simulink model "acvh_tuner"  (R2020b)
settings: Solver=VariableStepAuto  StartTime=0.0  StopTime=100  RelTol=1e-3
model workspace (MAT data in the model file):
  Var = 0
values from neighbouring files (symbols this model uses):
  dragCoeffMov = 0.01    [iris_quadcopter_specs.m]
  g = 9.81    [iris_quadcopter_specs.m]
  inertia = diag([Ixx, Iyy, Izz])    [iris_quadcopter_specs.m]
  mass = 0.8    [iris_quadcopter_specs.m]
  rotorDir = [-1, -1, 1, 1]    [iris_quadcopter_specs.m]
  rotorPositions = zeros(3,4)    [iris_quadcopter_specs.m]
  rotorThrustMax = 4    [iris_quadcopter_specs.m]
  rotorTimeConst = 0.005    [iris_quadcopter_specs.m]
  rotorTorqueMax = 0.05    [iris_quadcopter_specs.m]
  SampleTime = 0.001    [iris_quadcopter_specs.m]
  windVel = [0 0 0]'    [iris_quadcopter_specs.m]
undefined symbols (not defined in the file or in its folder): dev, DiscIntNeverNeededParam, Main, pwm_output0
libraries: pid_lib x6, shared6dof x5, simulink x3, shared6dofsys x2, px4lib x1, sharedtransform x1, sharedutil x1, px4uORBlib x1
settings Model: EnablePacing=on  Creator=sid  LastModifiedBy=sid

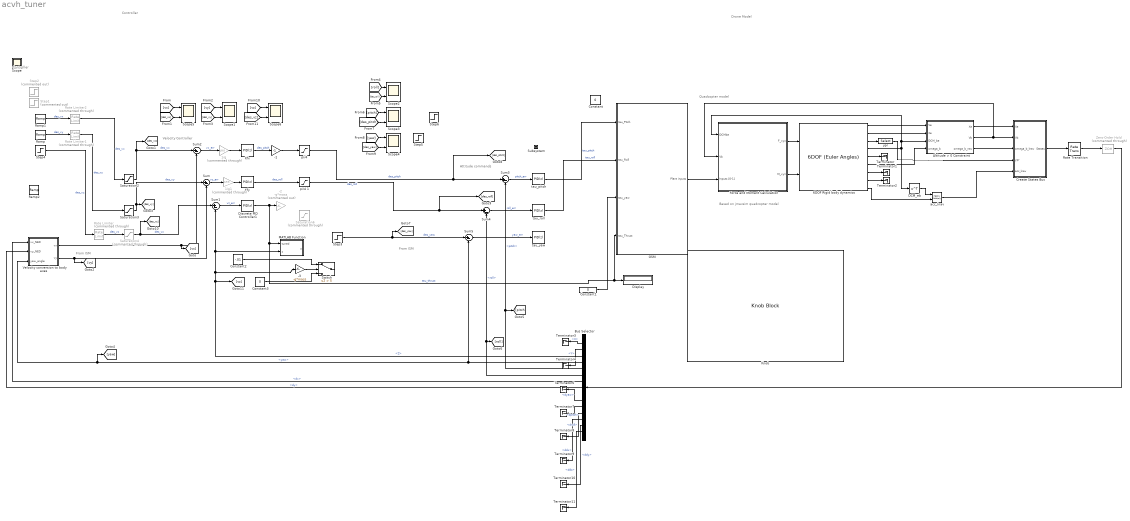
== system acvh_tuner ==
  note: Velocity Controller
  note: Attitude commands
  note: Controller
  note: Based on jmavsim quadcopter model
  note: Quadcopter model
  note: From ISM
  note: From ISM
  note: Controller
  note: Drone Model
  -1 : Gain  Gain=-1
  -2 : Gain  Commented=on  Gain=-g*mass
  -3 : Gain  Gain=-g*mass
  1/g : Gain  Commented=through  Gain=1/9.8
  1/g1 : Gain  Commented=through  Gain=1/9.8
  "6DOF Rigid body dynamics " : shared6dof/6DOF (Euler Angles)  units=Metric (MKS)  mtype=Fixed  rep=Euler Angles  xme_0=init.posNED  Vm_0=init.vb  eul_0=init.euler  pm_0=init.angRates  mass_0=mass  mass_e=0.5  mass_f=2.0  inertia=inertia  inertia_e=eye(3)  inertia_f=2*eye(3)  k_quat=Vehicle.SixDOF.quatGain  vre_flag=on  abi_flag=on  aMode=aMode  xme_statename=''  Vm_statename=''  eul_statename=''  quat_statename=''  pm_statename=''  mass_statename=''
      settings: SourceProductBaseCode=AE,PW,MT,UV,VE,VP
  Altitude > 0 Constraint : MATLAB Function  TreatAsAtomicUnit=on
  Bus Selector : BusSelector  OutputSignals=X,Y,Z,yaw,pitch,roll,dx,dy,dz,dyaw,dpitch,droll,ddx,ddy,ddz
  Constant : Constant  Value=0  SampleTime=SampleTime
  Constant1 : Constant  Value=0  SampleTime=SampleTime
  Constant2 : Constant  Value=-.01  SampleTime=SampleTime
  Constant3 : Constant  Value=0  SampleTime=SampleTime
  Create States Bus : Subsystem
  DCM_eb : Math  Operator=transpose  SaturateOnIntegerOverflow=on
  Discrete PID Controller1 : pid_lib/PID Controller  Controller=PID  Form=Parallel  TimeDomain=Discrete-time  UseExternalTs=off  SampleTime=SampleTime  IntegratorMethod=Trapezoidal  FilterMethod=Trapezoidal  ControllerParametersSource=internal  P=-0.0534535340221691  I=-0.00566953766767209  D=-0.123220888476467  UseFilter=on  N=26.3491959083223  TunerSelectOption=Transfer Function Based (PID Tuner App)  InitialConditionSource=internal  InitialConditionForIntegrator=0  InitialConditionForFilter=0  DifferentiatorICPrevScaledInput=0  ExternalReset=none  TrackingMode=off  Kt=1  LimitOutput=off  SatLimitsSource=internal  UpperSaturationLimit=10  LowerSaturationLimit=-.05  LinearizeAsGain=off  AntiWindupMode=back-calculation  Kb=10  POutMin=[]  POutMax=[]  IOutMin=[]  IOutMax=[]  DOutMin=[]  DOutMax=[]  NOutMin=[]  NOutMax=[]  SumOutMin=[]  SumOutMax=[]  SaturationOutMin=[]  SaturationOutMax=[]  PParamMin=[]  PParamMax=[]  IParamMin=[]  IParamMax=[]  DParamMin=[]  DParamMax=[]  NParamMin=[]  NParamMax=[]  KbParamMin=[]  KbParamMax=[]  KtParamMin=[]  KtParamMax=[]  KbOutMin=[]  KbOutMax=[]  KtOutMin=[]  KtOutMax=[]  IntegratorOutMin=[]  IntegratorOutMax=[]  FilterOutMin=[]  FilterOutMax=[]  SumI1OutMin=[]  SumI1OutMax=[]  SumI2OutMin=[]  SumI2OutMax=[]  SumI3OutMin=[]  SumI3OutMax=[]  SumI4OutMin=[]  SumI4OutMax=[]  SumDOutMin=[]  SumDOutMax=[]  DifferentiatorOutMin=[]  DifferentiatorOutMax=[]  FilterDiffOutCoefMin=[]  FilterDiffOutCoefMax=[]  ReciprocalOutMin=[]  ReciprocalOutMax=[]  SumDenOutMin=[]  SumDenOutMax=[]  SumNumOutMin=[]  SumNumOutMax=[]  DivideOutMin=[]  DivideOutMax=[]  UdiffTsProdOutMin=[]  UdiffTsProdOutMax=[]  NTsProdOutMin=[]  NTsProdOutMax=[]  UintegralTsProdOutMin=[]  UintegralTsProdOutMax=[]  UngainTsProdOutMin=[]  UngainTsProdOutMax=[]  IntegratorContinuousStateAttributes=''  IntegratorStateMustResolveToSignalObject=off  IntegratorRTWStateStorageClass=Auto  FilterContinuousStateAttributes=''  FilterStateMustResolveToSignalObject=off  FilterRTWStateStorageClass=Auto  ParallelPVariant=InternalParameters  IdealPVariant=Disabled  IVariant=InternalParameters  DVariant=InternalParameters  IntegratorVariant=Discrete  SatVariant=Disabled  AWVariant=Passthrough  PCopyVariant=Disabled  TRVariant=Disabled  FdbkBlocksVariant=Forward  IdealPFdbkVariant=Disabled  SatFdbkVariant=Disabled  DerivativeFilterVariant=TrapezoidalFilter  NVariant=InternalParameters  NCopyVariant=InternalParameters  FilterICVariant=InternalICsFilter  IntegratorICVariant=InternalICs  ExternalResetVariant=Disabled  TRSumVariant=Passthrough  SumFdbkVariant=Disabled  SumVariant=Sum_PID  TsampFilterVariant=InternalTs  TsampNgainVariant=Passthrough  TsampIntegralVariant=Passthrough  ExternalSaturationOutDataTypeStr=Inherit: Same as second input
  Display : Display
  Force and Moment Calculation : Subsystem
  Kfx : pid_lib/PID Controller  Controller=PID  Form=Parallel  TimeDomain=Discrete-time  UseExternalTs=off  SampleTime=SampleTime  IntegratorMethod=Forward Euler  FilterMethod=Forward Euler  ControllerParametersSource=internal  P=0.183358617742533  I=0.0739424315877928  D=-0.024031657470412  UseFilter=on  N=7.50922781087257  TunerSelectOption=Transfer Function Based (PID Tuner App)  InitialConditionSource=internal  InitialConditionForIntegrator=0  InitialConditionForFilter=0  DifferentiatorICPrevScaledInput=0  ExternalReset=none  TrackingMode=off  Kt=1  LimitOutput=on  SatLimitsSource=internal  UpperSaturationLimit=pi/8  LowerSaturationLimit=-pi/8  LinearizeAsGain=off  AntiWindupMode=clamping  Kb=1  POutMin=[]  POutMax=[]  IOutMin=[]  IOutMax=[]  DOutMin=[]  DOutMax=[]  NOutMin=[]  NOutMax=[]  SumOutMin=[]  SumOutMax=[]  SaturationOutMin=[]  SaturationOutMax=[]  PParamMin=[]  PParamMax=[]  IParamMin=[]  IParamMax=[]  DParamMin=[]  DParamMax=[]  NParamMin=[]  NParamMax=[]  KbParamMin=[]  KbParamMax=[]  KtParamMin=[]  KtParamMax=[]  KbOutMin=[]  KbOutMax=[]  KtOutMin=[]  KtOutMax=[]  IntegratorOutMin=[]  IntegratorOutMax=[]  FilterOutMin=[]  FilterOutMax=[]  SumI1OutMin=[]  SumI1OutMax=[]  SumI2OutMin=[]  SumI2OutMax=[]  SumI3OutMin=[]  SumI3OutMax=[]  SumI4OutMin=[]  SumI4OutMax=[]  SumDOutMin=[]  SumDOutMax=[]  DifferentiatorOutMin=[]  DifferentiatorOutMax=[]  FilterDiffOutCoefMin=[]  FilterDiffOutCoefMax=[]  ReciprocalOutMin=[]  ReciprocalOutMax=[]  SumDenOutMin=[]  SumDenOutMax=[]  SumNumOutMin=[]  SumNumOutMax=[]  DivideOutMin=[]  DivideOutMax=[]  UdiffTsProdOutMin=[]  UdiffTsProdOutMax=[]  NTsProdOutMin=[]  NTsProdOutMax=[]  UintegralTsProdOutMin=[]  UintegralTsProdOutMax=[]  UngainTsProdOutMin=[]  UngainTsProdOutMax=[]  IntegratorContinuousStateAttributes=''  IntegratorStateMustResolveToSignalObject=off  IntegratorRTWStateStorageClass=Auto  FilterContinuousStateAttributes=''  FilterStateMustResolveToSignalObject=off  FilterRTWStateStorageClass=Auto  ParallelPVariant=InternalParameters  IdealPVariant=Disabled  IVariant=InternalParameters  DVariant=InternalParameters  IntegratorVariant=Discrete  SatVariant=Enabled  AWVariant=DiscClampingParallel  PCopyVariant=Disabled  TRVariant=Disabled  FdbkBlocksVariant=Forward  IdealPFdbkVariant=Disabled  SatFdbkVariant=Disabled  DerivativeFilterVariant=ForwardEulerFilter  NVariant=InternalParameters  NCopyVariant=Disabled  FilterICVariant=InternalICsFilter  IntegratorICVariant=InternalICs  ExternalResetVariant=Disabled  TRSumVariant=Passthrough  SumFdbkVariant=Disabled  SumVariant=Sum_PID  TsampFilterVariant=InternalTs  TsampNgainVariant=Passthrough  TsampIntegralVariant=Passthrough  ExternalSaturationOutDataTypeStr=Inherit: Same as second input
  Kfy : pid_lib/PID Controller  Controller=PID  Form=Parallel  TimeDomain=Discrete-time  UseExternalTs=off  SampleTime=SampleTime  IntegratorMethod=Forward Euler  FilterMethod=Forward Euler  ControllerParametersSource=internal  P=0.183358617742446  I=0.0739424315877666  D=-0.0240316574704006  UseFilter=on  N=7.50922781087257  TunerSelectOption=Transfer Function Based (PID Tuner App)  InitialConditionSource=internal  InitialConditionForIntegrator=0  InitialConditionForFilter=0  DifferentiatorICPrevScaledInput=0  ExternalReset=none  TrackingMode=off  Kt=1  LimitOutput=on  SatLimitsSource=internal  UpperSaturationLimit=pi/8  LowerSaturationLimit=-pi/8  LinearizeAsGain=off  AntiWindupMode=clamping  Kb=1  POutMin=[]  POutMax=[]  IOutMin=[]  IOutMax=[]  DOutMin=[]  DOutMax=[]  NOutMin=[]  NOutMax=[]  SumOutMin=[]  SumOutMax=[]  SaturationOutMin=[]  SaturationOutMax=[]  PParamMin=[]  PParamMax=[]  IParamMin=[]  IParamMax=[]  DParamMin=[]  DParamMax=[]  NParamMin=[]  NParamMax=[]  KbParamMin=[]  KbParamMax=[]  KtParamMin=[]  KtParamMax=[]  KbOutMin=[]  KbOutMax=[]  KtOutMin=[]  KtOutMax=[]  IntegratorOutMin=[]  IntegratorOutMax=[]  FilterOutMin=[]  FilterOutMax=[]  SumI1OutMin=[]  SumI1OutMax=[]  SumI2OutMin=[]  SumI2OutMax=[]  SumI3OutMin=[]  SumI3OutMax=[]  SumI4OutMin=[]  SumI4OutMax=[]  SumDOutMin=[]  SumDOutMax=[]  DifferentiatorOutMin=[]  DifferentiatorOutMax=[]  FilterDiffOutCoefMin=[]  FilterDiffOutCoefMax=[]  ReciprocalOutMin=[]  ReciprocalOutMax=[]  SumDenOutMin=[]  SumDenOutMax=[]  SumNumOutMin=[]  SumNumOutMax=[]  DivideOutMin=[]  DivideOutMax=[]  UdiffTsProdOutMin=[]  UdiffTsProdOutMax=[]  NTsProdOutMin=[]  NTsProdOutMax=[]  UintegralTsProdOutMin=[]  UintegralTsProdOutMax=[]  UngainTsProdOutMin=[]  UngainTsProdOutMax=[]  IntegratorContinuousStateAttributes=''  IntegratorStateMustResolveToSignalObject=off  IntegratorRTWStateStorageClass=Auto  FilterContinuousStateAttributes=''  FilterStateMustResolveToSignalObject=off  FilterRTWStateStorageClass=Auto  ParallelPVariant=InternalParameters  IdealPVariant=Disabled  IVariant=InternalParameters  DVariant=InternalParameters  IntegratorVariant=Discrete  SatVariant=Enabled  AWVariant=DiscClampingParallel  PCopyVariant=Disabled  TRVariant=Disabled  FdbkBlocksVariant=Forward  IdealPFdbkVariant=Disabled  SatFdbkVariant=Disabled  DerivativeFilterVariant=ForwardEulerFilter  NVariant=InternalParameters  NCopyVariant=Disabled  FilterICVariant=InternalICsFilter  IntegratorICVariant=InternalICs  ExternalResetVariant=Disabled  TRSumVariant=Passthrough  SumFdbkVariant=Disabled  SumVariant=Sum_PID  TsampFilterVariant=InternalTs  TsampNgainVariant=Passthrough  TsampIntegralVariant=Passthrough  ExternalSaturationOutDataTypeStr=Inherit: Same as second input
  Knob : KnobBlock  ScaleMin=-1  ScaleMax=0
  MATLAB Function : MATLAB Function  TreatAsAtomicUnit=on
  OSM : Subsystem
  Ramp : simulink/Sources/Ramp  slope=3  start=10  InitialOutput=0
  Ramp1 : simulink/Sources/Ramp  slope=3  start=40  InitialOutput=0
  Ramp2 : simulink/Sources/Ramp  slope=-0.5  start=0  InitialOutput=-5
  Rate Limiter : RateLimiter  Commented=through  RisingSlewLimit=3  FallingSlewLimit=-3  SampleTimeMode=inherited  InitialCondition=-5
  Rate Limiter1 : RateLimiter  Commented=through  RisingSlewLimit=3  FallingSlewLimit=-3
  Rate Limiter2 : RateLimiter  Commented=through  RisingSlewLimit=3  FallingSlewLimit=-3
  Rate Transition : RateTransition  OutPortSampleTime=SampleTime
  Saturation2 : Saturate  UpperLimit=8  LowerLimit=-8  LinearizeAsGain=off
  Saturation3 : Saturate  UpperLimit=8  LowerLimit=-8  LinearizeAsGain=off
  Saturation4 : Saturate  Commented=through  UpperLimit=1  LowerLimit=-6
  Saturation6 : Saturate  Commented=through  UpperLimit=.12*g*mass  LowerLimit=-5*g*mass  SampleTime=SampleTime
  Scope{1..6} (6 alike) : Scope  NumInputPorts=2
  Step1 : Step  Commented=on  Time=40  SampleTime=SampleTime
  Step2 : Step  Commented=on  Time=10  SampleTime=SampleTime
  Step3 : Step  SampleTime=SampleTime
  Step4 : Step  Before=-5  After=-6  SampleTime=SampleTime
  Step5 : Step  After=pi/5  SampleTime=SampleTime
  Step6 : Step  After=pi/5  SampleTime=SampleTime
  Subsystem : Subsystem
  Sum{,1..5} (6 alike) : Sum  Inputs=|+-
  Switch : Switch  Criteria=u2 > Threshold  Threshold=5
  Terminator{,1..4,6..11} (11 alike) : Terminator
  Velocity conversion to body axes : Subsystem
  Zero-Order Hold : ZeroOrderHold  Commented=through  SampleTime=SampleTime
  acc_lnav : Product  Multiplication=Matrix(*)
  pi/4 : Saturate  UpperLimit=pi/4  LowerLimit=-pi/4
  pi/4 1 : Saturate  UpperLimit=pi/4  LowerLimit=-pi/4
  tau_pitch : pid_lib/PID Controller  Controller=PID  Form=Parallel  TimeDomain=Discrete-time  UseExternalTs=off  SampleTime=SampleTime  IntegratorMethod=Forward Euler  FilterMethod=Forward Euler  ControllerParametersSource=internal  P=0.0543673511512337  I=0.0109980209644375  D=0.0263229670839572  UseFilter=on  N=347.83750102845  TunerSelectOption=Transfer Function Based (PID Tuner App)  InitialConditionSource=internal  InitialConditionForIntegrator=0  InitialConditionForFilter=0  DifferentiatorICPrevScaledInput=0  ExternalReset=none  TrackingMode=off  Kt=1  LimitOutput=on  SatLimitsSource=internal  UpperSaturationLimit=.05  LowerSaturationLimit=-.05  LinearizeAsGain=off  AntiWindupMode=none  Kb=1  POutMin=[]  POutMax=[]  IOutMin=[]  IOutMax=[]  DOutMin=[]  DOutMax=[]  NOutMin=[]  NOutMax=[]  SumOutMin=[]  SumOutMax=[]  SaturationOutMin=[]  SaturationOutMax=[]  PParamMin=[]  PParamMax=[]  IParamMin=[]  IParamMax=[]  DParamMin=[]  DParamMax=[]  NParamMin=[]  NParamMax=[]  KbParamMin=[]  KbParamMax=[]  KtParamMin=[]  KtParamMax=[]  KbOutMin=[]  KbOutMax=[]  KtOutMin=[]  KtOutMax=[]  IntegratorOutMin=[]  IntegratorOutMax=[]  FilterOutMin=[]  FilterOutMax=[]  SumI1OutMin=[]  SumI1OutMax=[]  SumI2OutMin=[]  SumI2OutMax=[]  SumI3OutMin=[]  SumI3OutMax=[]  SumI4OutMin=[]  SumI4OutMax=[]  SumDOutMin=[]  SumDOutMax=[]  DifferentiatorOutMin=[]  DifferentiatorOutMax=[]  FilterDiffOutCoefMin=[]  FilterDiffOutCoefMax=[]  ReciprocalOutMin=[]  ReciprocalOutMax=[]  SumDenOutMin=[]  SumDenOutMax=[]  SumNumOutMin=[]  SumNumOutMax=[]  DivideOutMin=[]  DivideOutMax=[]  UdiffTsProdOutMin=[]  UdiffTsProdOutMax=[]  NTsProdOutMin=[]  NTsProdOutMax=[]  UintegralTsProdOutMin=[]  UintegralTsProdOutMax=[]  UngainTsProdOutMin=[]  UngainTsProdOutMax=[]  IntegratorContinuousStateAttributes=''  IntegratorStateMustResolveToSignalObject=off  IntegratorRTWStateStorageClass=Auto  FilterContinuousStateAttributes=''  FilterStateMustResolveToSignalObject=off  FilterRTWStateStorageClass=Auto  ParallelPVariant=InternalParameters  IdealPVariant=Disabled  IVariant=InternalParameters  DVariant=InternalParameters  IntegratorVariant=Discrete  SatVariant=Enabled  AWVariant=Passthrough  PCopyVariant=Disabled  TRVariant=Disabled  FdbkBlocksVariant=Forward  IdealPFdbkVariant=Disabled  SatFdbkVariant=Disabled  DerivativeFilterVariant=ForwardEulerFilter  NVariant=InternalParameters  NCopyVariant=Disabled  FilterICVariant=InternalICsFilter  IntegratorICVariant=InternalICs  ExternalResetVariant=Disabled  TRSumVariant=Passthrough  SumFdbkVariant=Disabled  SumVariant=Sum_PID  TsampFilterVariant=InternalTs  TsampNgainVariant=Passthrough  TsampIntegralVariant=Passthrough  ExternalSaturationOutDataTypeStr=Inherit: Same as second input
  tau_roll : pid_lib/PID Controller  Controller=PID  Form=Parallel  TimeDomain=Discrete-time  UseExternalTs=off  SampleTime=SampleTime  IntegratorMethod=Forward Euler  FilterMethod=Forward Euler  ControllerParametersSource=internal  P=-0.0543673511512337  I=-0.0109980209644375  D=-0.0263229670839572  UseFilter=on  N=347.83750102845  TunerSelectOption=Transfer Function Based (PID Tuner App)  InitialConditionSource=internal  InitialConditionForIntegrator=0  InitialConditionForFilter=0  DifferentiatorICPrevScaledInput=0  ExternalReset=none  TrackingMode=off  Kt=1  LimitOutput=on  SatLimitsSource=internal  UpperSaturationLimit=.05  LowerSaturationLimit=-.05  LinearizeAsGain=off  AntiWindupMode=none  Kb=1  POutMin=[]  POutMax=[]  IOutMin=[]  IOutMax=[]  DOutMin=[]  DOutMax=[]  NOutMin=[]  NOutMax=[]  SumOutMin=[]  SumOutMax=[]  SaturationOutMin=[]  SaturationOutMax=[]  PParamMin=[]  PParamMax=[]  IParamMin=[]  IParamMax=[]  DParamMin=[]  DParamMax=[]  NParamMin=[]  NParamMax=[]  KbParamMin=[]  KbParamMax=[]  KtParamMin=[]  KtParamMax=[]  KbOutMin=[]  KbOutMax=[]  KtOutMin=[]  KtOutMax=[]  IntegratorOutMin=[]  IntegratorOutMax=[]  FilterOutMin=[]  FilterOutMax=[]  SumI1OutMin=[]  SumI1OutMax=[]  SumI2OutMin=[]  SumI2OutMax=[]  SumI3OutMin=[]  SumI3OutMax=[]  SumI4OutMin=[]  SumI4OutMax=[]  SumDOutMin=[]  SumDOutMax=[]  DifferentiatorOutMin=[]  DifferentiatorOutMax=[]  FilterDiffOutCoefMin=[]  FilterDiffOutCoefMax=[]  ReciprocalOutMin=[]  ReciprocalOutMax=[]  SumDenOutMin=[]  SumDenOutMax=[]  SumNumOutMin=[]  SumNumOutMax=[]  DivideOutMin=[]  DivideOutMax=[]  UdiffTsProdOutMin=[]  UdiffTsProdOutMax=[]  NTsProdOutMin=[]  NTsProdOutMax=[]  UintegralTsProdOutMin=[]  UintegralTsProdOutMax=[]  UngainTsProdOutMin=[]  UngainTsProdOutMax=[]  IntegratorContinuousStateAttributes=''  IntegratorStateMustResolveToSignalObject=off  IntegratorRTWStateStorageClass=Auto  FilterContinuousStateAttributes=''  FilterStateMustResolveToSignalObject=off  FilterRTWStateStorageClass=Auto  ParallelPVariant=InternalParameters  IdealPVariant=Disabled  IVariant=InternalParameters  DVariant=InternalParameters  IntegratorVariant=Discrete  SatVariant=Enabled  AWVariant=Passthrough  PCopyVariant=Disabled  TRVariant=Disabled  FdbkBlocksVariant=Forward  IdealPFdbkVariant=Disabled  SatFdbkVariant=Disabled  DerivativeFilterVariant=ForwardEulerFilter  NVariant=InternalParameters  NCopyVariant=Disabled  FilterICVariant=InternalICsFilter  IntegratorICVariant=InternalICs  ExternalResetVariant=Disabled  TRSumVariant=Passthrough  SumFdbkVariant=Disabled  SumVariant=Sum_PID  TsampFilterVariant=InternalTs  TsampNgainVariant=Passthrough  TsampIntegralVariant=Passthrough  ExternalSaturationOutDataTypeStr=Inherit: Same as second input
  tau_yaw : pid_lib/PID Controller  Controller=PID  Form=Parallel  TimeDomain=Discrete-time  UseExternalTs=off  SampleTime=SampleTime  IntegratorMethod=Forward Euler  FilterMethod=Forward Euler  ControllerParametersSource=internal  P=-0.564155915391973  I=-0.130215223566003  D=-0.447814603729917  UseFilter=on  N=347.83750102845  TunerSelectOption=Transfer Function Based (PID Tuner App)  InitialConditionSource=internal  InitialConditionForIntegrator=0  InitialConditionForFilter=0  DifferentiatorICPrevScaledInput=0  ExternalReset=none  TrackingMode=off  Kt=1  LimitOutput=on  SatLimitsSource=internal  UpperSaturationLimit=0.1  LowerSaturationLimit=-0.1  LinearizeAsGain=off  AntiWindupMode=none  Kb=1  POutMin=[]  POutMax=[]  IOutMin=[]  IOutMax=[]  DOutMin=[]  DOutMax=[]  NOutMin=[]  NOutMax=[]  SumOutMin=[]  SumOutMax=[]  SaturationOutMin=[]  SaturationOutMax=[]  PParamMin=[]  PParamMax=[]  IParamMin=[]  IParamMax=[]  DParamMin=[]  DParamMax=[]  NParamMin=[]  NParamMax=[]  KbParamMin=[]  KbParamMax=[]  KtParamMin=[]  KtParamMax=[]  KbOutMin=[]  KbOutMax=[]  KtOutMin=[]  KtOutMax=[]  IntegratorOutMin=[]  IntegratorOutMax=[]  FilterOutMin=[]  FilterOutMax=[]  SumI1OutMin=[]  SumI1OutMax=[]  SumI2OutMin=[]  SumI2OutMax=[]  SumI3OutMin=[]  SumI3OutMax=[]  SumI4OutMin=[]  SumI4OutMax=[]  SumDOutMin=[]  SumDOutMax=[]  DifferentiatorOutMin=[]  DifferentiatorOutMax=[]  FilterDiffOutCoefMin=[]  FilterDiffOutCoefMax=[]  ReciprocalOutMin=[]  ReciprocalOutMax=[]  SumDenOutMin=[]  SumDenOutMax=[]  SumNumOutMin=[]  SumNumOutMax=[]  DivideOutMin=[]  DivideOutMax=[]  UdiffTsProdOutMin=[]  UdiffTsProdOutMax=[]  NTsProdOutMin=[]  NTsProdOutMax=[]  UintegralTsProdOutMin=[]  UintegralTsProdOutMax=[]  UngainTsProdOutMin=[]  UngainTsProdOutMax=[]  IntegratorContinuousStateAttributes=''  IntegratorStateMustResolveToSignalObject=off  IntegratorRTWStateStorageClass=Auto  FilterContinuousStateAttributes=''  FilterStateMustResolveToSignalObject=off  FilterRTWStateStorageClass=Auto  ParallelPVariant=InternalParameters  IdealPVariant=Disabled  IVariant=InternalParameters  DVariant=InternalParameters  IntegratorVariant=Discrete  SatVariant=Enabled  AWVariant=Passthrough  PCopyVariant=Disabled  TRVariant=Disabled  FdbkBlocksVariant=Forward  IdealPFdbkVariant=Disabled  SatFdbkVariant=Disabled  DerivativeFilterVariant=ForwardEulerFilter  NVariant=InternalParameters  NCopyVariant=Disabled  FilterICVariant=InternalICsFilter  IntegratorICVariant=InternalICs  ExternalResetVariant=Disabled  TRSumVariant=Passthrough  SumFdbkVariant=Disabled  SumVariant=Sum_PID  TsampFilterVariant=InternalTs  TsampNgainVariant=Passthrough  TsampIntegralVariant=Passthrough  ExternalSaturationOutDataTypeStr=Inherit: Same as second input
  ypr : Selector  InputPortWidth=3  IndexOptions=Index vector (dialog)  Indices=[3 2 1]  OutputSizes=1
  Scope : Scope
  wires:
  "6DOF Rigid body dynamics "/6 -> Altitude > 0 Constraint/4(omega_b)
  Altitude > 0 Constraint/1(Xe) -> Create States Bus/1(Xe)
  "6DOF Rigid body dynamics "/1 -> Altitude > 0 Constraint/1(Ve)
  "6DOF Rigid body dynamics "/2 -> Altitude > 0 Constraint/2("Xe ")
  "6DOF Rigid body dynamics "/3 -> ypr/1
  acc_lnav/1 -> Create States Bus/5(acc_lnav)
  "6DOF Rigid body dynamics "/5 -> Terminator/1
  Altitude > 0 Constraint/3(omega_b_nav) -> Create States Bus/3(omega_b_lnav)
  "6DOF Rigid body dynamics "/9 -> acc_lnav/2
  "6DOF Rigid body dynamics "/4 -> DCM_eb/1, Force and Moment Calculation/1(DCMbe), Altitude > 0 Constraint/3(DCM_be)
  DCM_eb/1 -> acc_lnav/1
  Force and Moment Calculation/2(M_xyz) -> "6DOF Rigid body dynamics "/2
  "6DOF Rigid body dynamics "/7 -> Terminator1/1
  "6DOF Rigid body dynamics "/8 -> Terminator2/1
  Force and Moment Calculation/1(F_xyz) -> "6DOF Rigid body dynamics "/1
  Create States Bus/1(States) -> Rate Transition/1
  ypr/1 -> Create States Bus/4(ypr)
  OSM/1(Plant inputs) -> Force and Moment Calculation/3(Inputs [0-1])
  Altitude > 0 Constraint/2(Vb) -> Force and Moment Calculation/2(Vb), Create States Bus/2(Vb)
  Zero-Order Hold/1 -> Bus Selector/1
  Bus Selector/1 -> Terminator3/1  "<X>"
  Bus Selector/2 -> Terminator4/1  "<Y>"
  Bus Selector/4 -> [yaw], Velocity conversion to body axes/3(yaw_angle), Sum5/2  "<yaw>"
  Bus Selector/5 -> [pitch], Sum3/2  "<pitch>"
  Bus Selector/6 -> Sum4/2, [roll]  "<roll>"
  Bus Selector/7 -> Velocity conversion to body axes/1(vx_NED)  "<dx>"
  Bus Selector/8 -> Velocity conversion to body axes/2(vy_NED)  "<dy>"
  Bus Selector/10 -> Terminator6/1  "<dyaw>"
  Bus Selector/11 -> Terminator7/1  "<dpitch>"
  Bus Selector/12 -> Terminator8/1  "<droll>"
  Bus Selector/13 -> Terminator9/1  "<ddx>"
  Bus Selector/14 -> Terminator10/1  "<ddy>"
  Bus Selector/15 -> Terminator11/1  "<ddz>"
  Rate Transition/1 -> Zero-Order Hold/1
  [des_yaw] -> Scope4/2
  [yaw] -> Scope4/1
  [des_pitch] -> Scope3/2
  [pitch] -> Scope3/1
  [des_roll] -> Scope2/2
  [roll] -> Scope2/1
  [des_vy] -> Scope1/2
  [vy] -> Scope1/1
  [des_vx] -> Scope5/2
  [vx] -> Scope5/1
  Step4/1 -> Rate Limiter/1  "des_vz"
  Sum3/1 -> tau_pitch/1  "pitch_err"
  Sum4/1 -> tau_roll/1  "roll_err"
  Sum5/1 -> tau_yaw/1  "yaw_err"
  Step3/1 -> [des_yaw], Sum5/1  "des_yaw"
  1/g1/1 -> Kfy/1
  1/g/1 -> Kfx/1
  Discrete PID Controller1/1 -> OSM/4(tau_Thrust), Display/1, MATLAB Function/1(tuned), -2/1  "tau_thrust"
  Velocity conversion to body axes/2(vy) -> Sum/2, [vy]
  Kfx/1 -> -1/1  "des_pitch"
  Saturation2/1 -> Sum2/1, [des_vx]  "des_vx"
  Velocity conversion to body axes/1(vx) -> Sum2/2, [vx]
  Sum/1 -> 1/g1/1  "vy_err"
  Saturation3/1 -> Sum/1, [des_vy]  "des_vy"
  Kfy/1 -> pi/4 1/1  "des_roll"
  Sum1/1 -> Discrete PID Controller1/1  "vz_err"
  Sum2/1 -> 1/g/1  "vx_err"
  -1/1 -> pi/4/1
  [vz] -> Scope6/1
  [des_vz] -> Scope6/2
  ? -> Subsystem/Trigger
  ? -> Subsystem/1(In1)
  pi/4/1 -> [des_pitch], Sum3/1  "des_pitch"
  pi/4 1/1 -> [des_roll], Sum4/1  "des_roll"
  Bus Selector/3 -> MATLAB Function/2(z), Sum1/2, -3/1, [vz]  "<Z>"
  Constant1/1 -> OSM/3(tau_yaw)
  Saturation4/1 -> Sum1/1, [des_vz]  "des_vz"
  tau_pitch/1 -> OSM/1(tau_Pitch)  "tau_pitch"
  tau_roll/1 -> OSM/2(tau_Roll)  "tau_roll"
  Rate Limiter/1 -> Saturation4/1  "des_vz"
  Rate Limiter1/1 -> Saturation3/1  "des_vy"
  Rate Limiter2/1 -> Saturation2/1  "des_vx"
  Ramp1/1 -> Rate Limiter2/1  "des_vx"
  Ramp/1 -> Rate Limiter1/1  "des_vy"
  -3/1 -> Switch/2
  Constant2/1 -> Switch/1
  Constant3/1 -> Switch/3

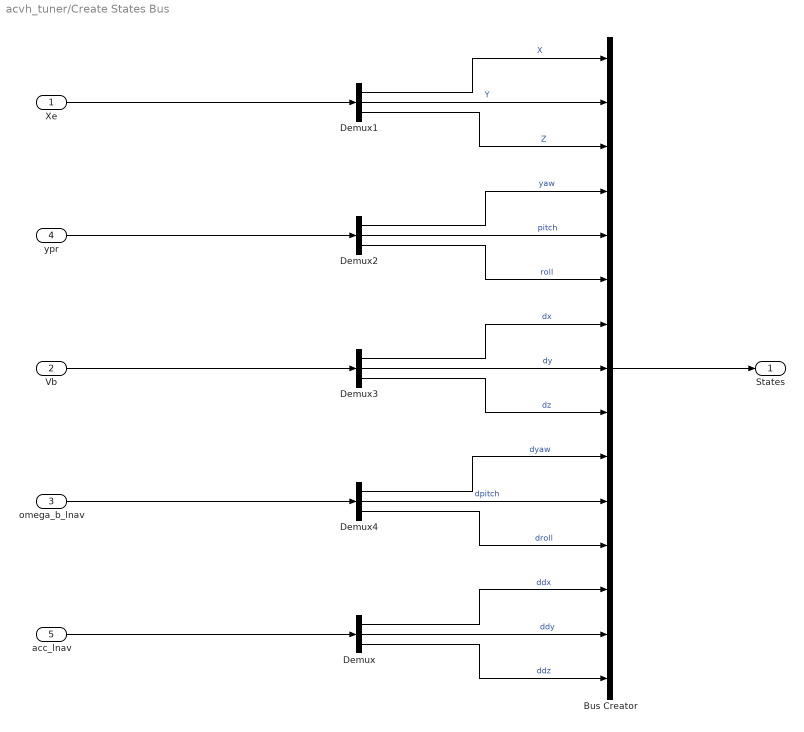
== system acvh_tuner/Create States Bus ==
  Xe : Inport
  Vb : Inport  Port=2
  omega_b_lnav : Inport  Port=3
  ypr : Inport  Port=4
  acc_lnav : Inport  Port=5
  Bus Creator : BusCreator  Inputs=15
  Demux{,1..4} (5 alike) : Demux  Outputs=3
  States : Outport
  wires:
  Demux1/1 -> Bus Creator/1  "X"
  Demux1/2 -> Bus Creator/2  "Y"
  ypr/1 -> Demux2/1
  Demux2/2 -> Bus Creator/5  "pitch"
  Demux3/2 -> Bus Creator/8  "dy"
  Demux2/3 -> Bus Creator/6  "roll"
  omega_b_lnav/1 -> Demux4/1
  Vb/1 -> Demux3/1
  Demux2/1 -> Bus Creator/4  "yaw"
  Demux1/3 -> Bus Creator/3  "Z"
  Demux3/1 -> Bus Creator/7  "dx"
  Demux4/2 -> Bus Creator/11  "dpitch"
  Demux3/3 -> Bus Creator/9  "dz"
  Demux4/3 -> Bus Creator/12  "droll"
  Demux4/1 -> Bus Creator/10  "dyaw"
  Bus Creator/1 -> States/1
  Xe/1 -> Demux1/1
  acc_lnav/1 -> Demux/1
  Demux/3 -> Bus Creator/15  "ddz"
  Demux/2 -> Bus Creator/14  "ddy"
  Demux/1 -> Bus Creator/13  "ddx"

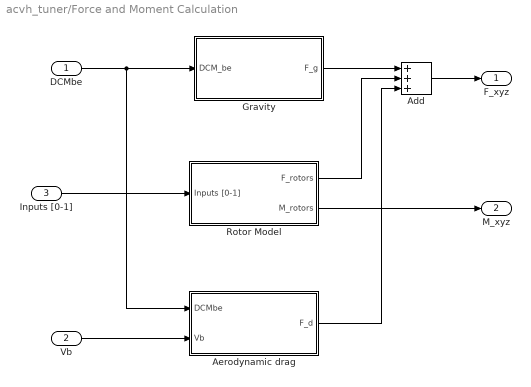
== system acvh_tuner/Force and Moment Calculation ==
  DCMbe : Inport
  Vb : Inport  Port=2
  Inputs [0-1] : Inport  Port=3
  Add : Sum  Inputs=+++
  Aerodynamic drag : Subsystem
  Gravity : Subsystem
  Rotor Model : Subsystem
  F_xyz : Outport
  M_xyz : Outport  Port=2
  wires:
  Inputs [0-1]/1 -> Rotor Model/1(Inputs [0-1])
  DCMbe/1 -> Aerodynamic drag/1(DCMbe), Gravity/1(DCM_be)
  Gravity/1(F_g) -> Add/1
  Add/1 -> F_xyz/1
  Rotor Model/2(M_rotors) -> M_xyz/1
  Vb/1 -> Aerodynamic drag/2(Vb)
  Rotor Model/1(F_rotors) -> Add/2
  Aerodynamic drag/1(F_d) -> Add/3

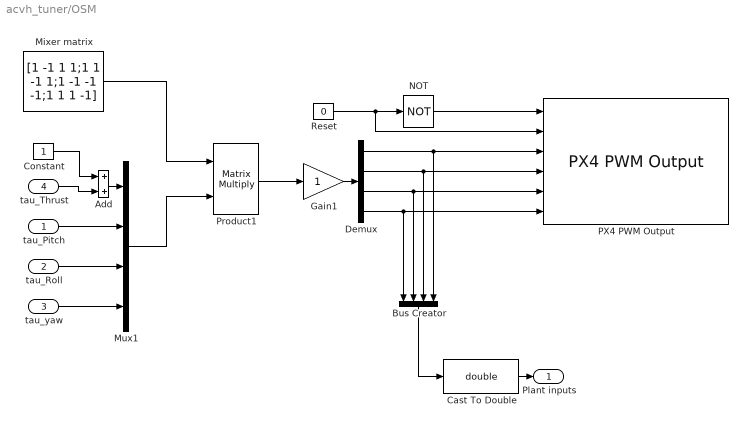
== system acvh_tuner/OSM ==
  tau_Pitch : Inport
  tau_Roll : Inport  Port=2
  tau_yaw : Inport  Port=3
  tau_Thrust : Inport  Port=4
  Add : Sum
  Bus Creator : BusCreator  Inputs=4
  Cast To Double : DataTypeConversion  OutDataTypeStr=double
  Constant : Constant  SampleTime=SampleTime
  Demux : Demux
  Gain1 : Gain  OutDataTypeStr=uint16
  Mixer matrix : Constant  Value=[1 -1 1 1;1 1 -1 1;1 -1 -1 -1;1 1 1 -1]  OutDataTypeStr=Inherit: Inherit via back propagation
  Mux1 : Mux
  NOT : Logic  Operator=NOT  IconShape=distinctive  AllPortsSameDT=off  OutDataTypeStr=boolean
  PX4 PWM Output : px4lib/PX4 PWM Output  pwmDevice=Main (/dev/pwm_output0)  pwmChannel1_=on  pwmChannel2_=on  pwmChannel3_=on  pwmChannel4_=on  pwmChannel5_=off  pwmChannel6_=off  pwmChannel7_=off  pwmChannel8_=off  forceTerminateFailsafe=off  outputErrorStatus=off
      settings: SourceProductBaseCode=PX4AUTOPILOTS
  Product1 : Product  Multiplication=Matrix(*)  RndMeth=Zero
  Reset : Constant  Value=0  OutDataTypeStr=boolean
  Plant inputs : Outport
  wires:
  NOT/1 -> PX4 PWM Output/1
  Mixer matrix/1 -> Product1/1
  tau_yaw/1 -> Mux1/4
  tau_Pitch/1 -> Mux1/2
  tau_Roll/1 -> Mux1/3
  Reset/1 -> PX4 PWM Output/2, NOT/1
  Demux/3 -> Bus Creator/2, PX4 PWM Output/5
  Demux/2 -> Bus Creator/3, PX4 PWM Output/4
  Mux1/1 -> Product1/2
  Demux/4 -> Bus Creator/1, PX4 PWM Output/6
  Gain1/1 -> Demux/1
  Demux/1 -> Bus Creator/4, PX4 PWM Output/3
  Product1/1 -> Gain1/1
  tau_Thrust/1 -> Add/2
  Add/1 -> Mux1/1
  Constant/1 -> Add/1
  Cast To Double/1 -> Plant inputs/1
  Bus Creator/1 -> Cast To Double/1

== system acvh_tuner/Subsystem ==
  In1 : Inport
  Trigger : TriggerPort  VariantControl=Variant  PortDimensions=1
  6DOF Rigid Body Dynamics : Subsystem  Commented=on
  Commands : Subsystem  Commented=on

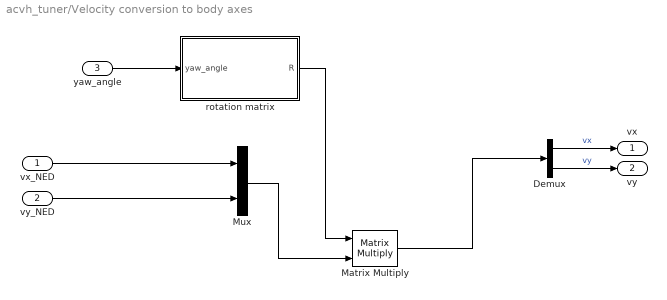
== system acvh_tuner/Velocity conversion to body axes ==
  vx_NED : Inport
  vy_NED : Inport  Port=2
  yaw_angle : Inport  Port=3
  Demux : Demux  Outputs=2
  Matrix Multiply : Product  Multiplication=Matrix(*)
  Mux : Mux  Inputs=2
  rotation matrix : Subsystem
  vx : Outport
  vy : Outport  Port=2
  wires:
  vy_NED/1 -> Mux/2
  vx_NED/1 -> Mux/1
  Demux/1 -> vx/1  "vx"
  Demux/2 -> vy/1  "vy"
  rotation matrix/1(R) -> Matrix Multiply/1
  Matrix Multiply/1 -> Demux/1
  yaw_angle/1 -> rotation matrix/1(yaw_angle)
  Mux/1 -> Matrix Multiply/2

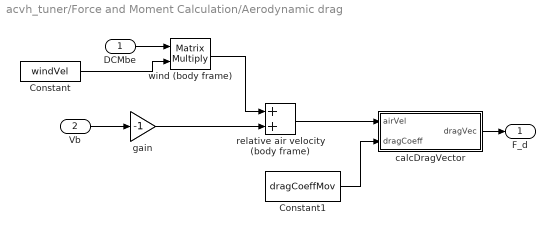
== system acvh_tuner/Force and Moment Calculation/Aerodynamic drag ==
  DCMbe : Inport
  Vb : Inport  Port=2
  Constant : Constant  Value=windVel  SampleTime=SampleTime
  Constant1 : Constant  Value=dragCoeffMov  SampleTime=SampleTime
  calcDragVector : MATLAB Function  TreatAsAtomicUnit=on
  gain : Gain  Gain=-1
  relative air velocity (body frame) : Sum
  wind (body frame) : Product  Multiplication=Matrix(*)
  F_d : Outport
  wires:
  Vb/1 -> gain/1
  calcDragVector/1(dragVec) -> F_d/1
  relative air velocity (body frame)/1 -> calcDragVector/1(airVel)
  gain/1 -> relative air velocity (body frame)/2
  Constant1/1 -> calcDragVector/2(dragCoeff)
  DCMbe/1 -> wind (body frame)/1
  Constant/1 -> wind (body frame)/2
  wind (body frame)/1 -> relative air velocity (body frame)/1

== system acvh_tuner/Force and Moment Calculation/Gravity ==
  DCM_be : Inport
  Constant : Constant  Value=[0 0 g]'
  Gain : Gain  Gain=mass
  Matrix Multiply : Product  Multiplication=Matrix(*)
  F_g : Outport
  wires:
  Matrix Multiply/1 -> Gain/1
  Constant/1 -> Matrix Multiply/2
  DCM_be/1 -> Matrix Multiply/1
  Gain/1 -> F_g/1

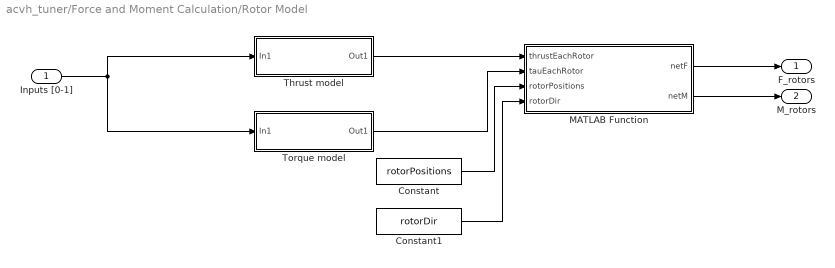
== system acvh_tuner/Force and Moment Calculation/Rotor Model ==
  Inputs [0-1] : Inport
  Constant : Constant  Value=rotorPositions
  Constant1 : Constant  Value=rotorDir
  MATLAB Function : MATLAB Function  TreatAsAtomicUnit=on
  Thrust model : Subsystem
  Torque model : Subsystem
  F_rotors : Outport
  M_rotors : Outport  Port=2
  wires:
  Inputs [0-1]/1 -> Torque model/1(In1), Thrust model/1(In1)
  MATLAB Function/1(netF) -> F_rotors/1
  MATLAB Function/2(netM) -> M_rotors/1
  Constant/1 -> MATLAB Function/3(rotorPositions)
  Constant1/1 -> MATLAB Function/4(rotorDir)
  Torque model/1(Out1) -> MATLAB Function/2(tauEachRotor)
  Thrust model/1(Out1) -> MATLAB Function/1(thrustEachRotor)

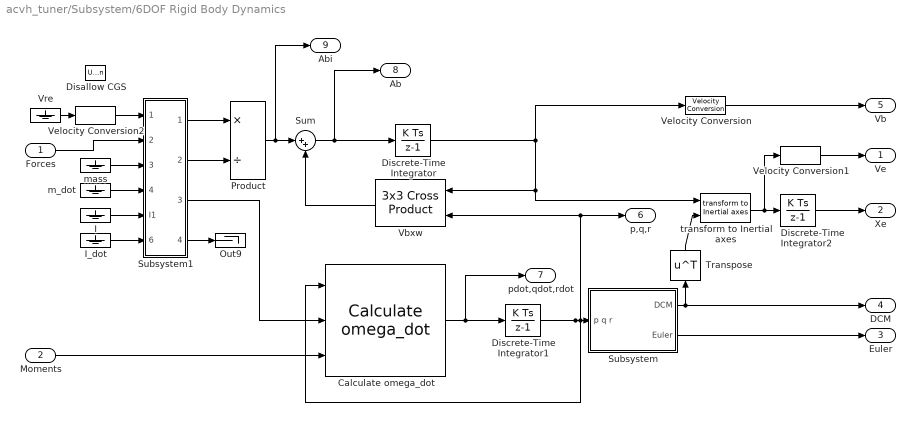
== system acvh_tuner/Subsystem/6DOF Rigid Body Dynamics ==
  Forces : Inport  Unit=N  PortDimensions=3
  Moments : Inport  Port=2  Unit=N*m  PortDimensions=3
  Calculate omega_dot : shared6dofsys/Calculate omega_dot  aMode=aMode
      settings: SourceProductBaseCode=AE,PW,MT,UV,VE,VP
  Disallow CGS : UnitConfiguration  UnitSystemsStr=English,SI,SI (extended)  AllowAllUnitSystems=off
  Discrete-Time Integrator : DiscreteIntegrator  SampleTime=SampleTime  ICPrevOutput=DiscIntNeverNeededParam  ICPrevScaledInput=DiscIntNeverNeededParam
  Discrete-Time Integrator1 : DiscreteIntegrator  SampleTime=SampleTime  ICPrevOutput=DiscIntNeverNeededParam  ICPrevScaledInput=DiscIntNeverNeededParam
  Discrete-Time Integrator2 : DiscreteIntegrator  SampleTime=SampleTime  ICPrevOutput=DiscIntNeverNeededParam  ICPrevScaledInput=DiscIntNeverNeededParam
  I : Ground
  I_dot : Ground
  Out9 : Terminator
  Product : Product  Inputs=*/  SaturateOnIntegerOverflow=on  OutDataTypeStr=Inherit: Same as first input
  Subsystem : Subsystem
  Subsystem1 : Subsystem
  Sum : Sum  Inputs=|++  SaturateOnIntegerOverflow=on
  Transpose : Math  Operator=transpose  SignedPower=on  SaturateOnIntegerOverflow=on
  Vbxw : sharedutil/3x3 Cross Product  aMode=aMode
      settings: SourceProductBaseCode=AE,PW,MT,UV,VE,VP
  Velocity Conversion : shared6dof/6DOF (Euler Angles)/Velocity Conversion  SystemSampleTime=-1  VariantActivationTime=update diagram  Latency=0  AutoFrameSizeCalculation=off
      settings: SourceProductBaseCode=AE,PW,MT,UV,VE,VP
  Velocity Conversion1 : shared6dof/6DOF (Euler Angles)/Velocity Conversion1  SystemSampleTime=-1  VariantActivationTime=update diagram  Latency=0  AutoFrameSizeCalculation=off
      settings: SourceProductBaseCode=AE,PW,MT,UV,VE,VP
  Velocity Conversion2 : shared6dof/6DOF (Euler Angles)/Velocity Conversion2  SystemSampleTime=-1  VariantActivationTime=update diagram  Latency=0  AutoFrameSizeCalculation=off
      settings: SourceProductBaseCode=AE,PW,MT,UV,VE,VP
  Vre : Ground
  m_dot : Ground
  mass : Ground
  "transform to Inertial axes " : shared6dof/6DOF (Euler Angles)/transform to Inertial axes   SystemSampleTime=-1  VariantActivationTime=update diagram  Latency=0  AutoFrameSizeCalculation=off
      settings: SourceProductBaseCode=AE,PW,MT,UV,VE,VP
  Ve : Outport  Unit=m/s  VectorParamsAs1DForOutWhenUnconnected=off
  Xe : Outport  Port=2  Unit=m  VectorParamsAs1DForOutWhenUnconnected=off
  Euler : Outport  Port=3  Unit=rad  VectorParamsAs1DForOutWhenUnconnected=off
  DCM : Outport  Port=4  Unit=1  VectorParamsAs1DForOutWhenUnconnected=off
  Vb : Outport  Port=5  Unit=m/s  VectorParamsAs1DForOutWhenUnconnected=off
  p,q,r : Outport  Port=6  Unit=rad/s  VectorParamsAs1DForOutWhenUnconnected=off
  pdot,qdot,rdot : Outport  Port=7  Unit=rad/s^2  VectorParamsAs1DForOutWhenUnconnected=off
  Ab : Outport  Port=8  Unit=m/s^2  VectorParamsAs1DForOutWhenUnconnected=off
  Abi : Outport  Port=9  Unit=m/s^2
  wires:
  mass/1 -> Subsystem1/3("mass ")
  Subsystem1/4(Out1) -> Out9/1
  Forces/1 -> Subsystem1/2(forces)
  Transpose/1 -> "transform to Inertial axes "/2
  Discrete-Time Integrator1/1 -> Calculate omega_dot/1, p,q,r/1, Vbxw/2, Subsystem/1("p q r ")
  Subsystem1/1("forces ") -> Product/1
  Discrete-Time Integrator2/1 -> Xe/1
  Vbxw/1 -> Sum/2
  "transform to Inertial axes "/1 -> Velocity Conversion1/1, Discrete-Time Integrator2/1
  Subsystem1/2(mass1) -> Product/2
  Velocity Conversion2/1 -> Subsystem1/1(Vre1)
  Calculate omega_dot/1 -> pdot,qdot,rdot/1, Discrete-Time Integrator1/1
  Velocity Conversion/1 -> Vb/1
  Product/1 -> Abi/1, Sum/1
  Sum/1 -> Ab/1, Discrete-Time Integrator/1
  m_dot/1 -> Subsystem1/4(m_dot1)
  Subsystem1/3("inertia, 0") -> Calculate omega_dot/2
  Discrete-Time Integrator/1 -> "transform to Inertial axes "/1, Vbxw/1, Velocity Conversion/1
  Subsystem/2(Euler) -> Euler/1
  Vre/1 -> Velocity Conversion2/1
  Moments/1 -> Calculate omega_dot/3
  Velocity Conversion1/1 -> Ve/1
  Subsystem/1(DCM) -> DCM/1, Transpose/1
  I_dot/1 -> Subsystem1/6(I_dot1)
  I/1 -> Subsystem1/5(I1)

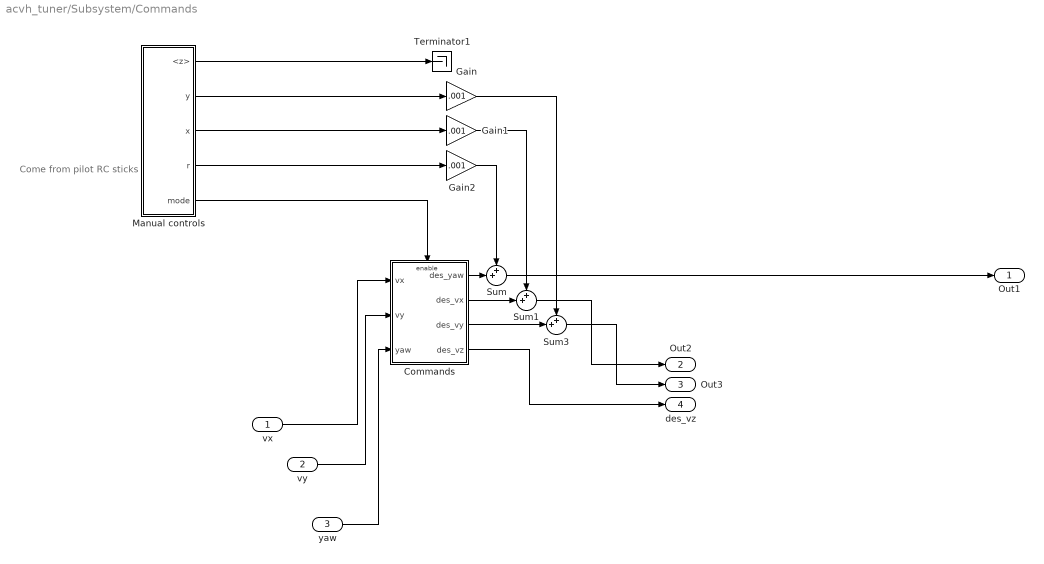
== system acvh_tuner/Subsystem/Commands ==
  note: Come from pilot RC sticks
  vx : Inport
  vy : Inport  Port=2
  yaw : Inport  Port=3
  "Commands " : Subsystem
  Gain : Gain  Gain=.001
  Gain1 : Gain  Gain=.001
  Gain2 : Gain  Gain=.001
  Manual controls : Subsystem
  Sum : Sum  Inputs=++|
  Sum1 : Sum  Inputs=++|
  Sum3 : Sum  Inputs=++|
  Terminator1 : Terminator
  Out1 : Outport
  Out2 : Outport  Port=2
  Out3 : Outport  Port=3
  des_vz : Outport  Port=4
  wires:
  Gain/1 -> Sum3/1
  "Commands "/4(des_vz) -> des_vz/1
  Manual controls/4(r) -> Gain2/1
  "Commands "/2(des_vx) -> Sum1/2
  Manual controls/5(mode) -> "Commands "/Enable
  Sum3/1 -> Out3/1
  "Commands "/1(des_yaw) -> Sum/2
  Manual controls/1(<z>) -> Terminator1/1
  Sum1/1 -> Out2/1
  Gain2/1 -> Sum/1
  Sum/1 -> Out1/1
  yaw/1 -> "Commands "/3(yaw)
  vy/1 -> "Commands "/2(vy)
  Manual controls/2(y) -> Gain/1
  "Commands "/3(des_vy) -> Sum3/2
  vx/1 -> "Commands "/1(vx)
  Manual controls/3(x) -> Gain1/1
  Gain1/1 -> Sum1/1

== system acvh_tuner/Velocity conversion to body axes/rotation matrix ==
  yaw_angle : Inport
  Gain : Gain  Gain=-1
  Matrix Concatenate : Concatenate  Mode=Multidimensional array  ConcatenateDimension=2
  Mux : Mux  Inputs=2
  Mux1 : Mux  Inputs=2
  Trigonometric Function : Trigonometry
  Trigonometric Function1 : Trigonometry  Operator=cos
  R : Outport
  wires:
  Mux1/1 -> Matrix Concatenate/2
  Trigonometric Function1/1 -> Mux1/2, Mux/1
  yaw_angle/1 -> Trigonometric Function1/1, Trigonometric Function/1
  Trigonometric Function/1 -> Gain/1, Mux1/1
  Mux/1 -> Matrix Concatenate/1
  Gain/1 -> Mux/2
  Matrix Concatenate/1 -> R/1

== system acvh_tuner/Force and Moment Calculation/Rotor Model/Thrust model ==
  In1 : Inport
  Demux : Demux
  Mux : Mux
  Transfer Fcn{,2..4} (4 alike) : TransferFcn  Numerator=[rotorThrustMax]  Denominator=[rotorTimeConst 1]
  Out1 : Outport
  wires:
  Transfer Fcn3/1 -> Mux/2
  Demux/1 -> Transfer Fcn4/1
  Transfer Fcn2/1 -> Mux/3
  Demux/3 -> Transfer Fcn2/1
  Mux/1 -> Out1/1
  Transfer Fcn4/1 -> Mux/1
  Demux/4 -> Transfer Fcn/1
  Demux/2 -> Transfer Fcn3/1
  Transfer Fcn/1 -> Mux/4
  In1/1 -> Demux/1

== system acvh_tuner/Force and Moment Calculation/Rotor Model/Torque model ==
  In1 : Inport
  Demux : Demux
  Mux : Mux
  Transfer Fcn{1..4} (4 alike) : TransferFcn  Numerator=[rotorTorqueMax]  Denominator=[rotorTimeConst 1]
  Out1 : Outport
  wires:
  Transfer Fcn4/1 -> Mux/4
  Demux/1 -> Transfer Fcn1/1
  Transfer Fcn3/1 -> Mux/3
  Transfer Fcn2/1 -> Mux/2
  Demux/2 -> Transfer Fcn2/1
  Demux/4 -> Transfer Fcn4/1
  Demux/3 -> Transfer Fcn3/1
  Mux/1 -> Out1/1
  Transfer Fcn1/1 -> Mux/1
  In1/1 -> Demux/1

== system acvh_tuner/Subsystem/6DOF Rigid Body Dynamics/Subsystem ==
  "p q r " : Inport
  Discrete-Time Integrator3 : DiscreteIntegrator  SampleTime=SampleTime  ICPrevOutput=DiscIntNeverNeededParam  ICPrevScaledInput=DiscIntNeverNeededParam
  Rotation Angles to Direction Cosine Matrix : sharedtransform/Rotation Angles to Direction Cosine Matrix  rotationOrder=ZYX  aMode=aMode
      settings: SourceProductBaseCode=AE,PW,MT,UV,VE,VP
  Selector : Selector  InputPortWidth=3  IndexOptions=Index vector (dialog)  Indices=[3 2 1]  OutputSizes=1
  phidot thetadot psidot : shared6dofsys/DCM & Euler Angles (Euler)/phidot thetadot psidot  SystemSampleTime=-1  VariantActivationTime=update diagram  Latency=0  AutoFrameSizeCalculation=off
      settings: SourceProductBaseCode=AE,PW,MT,UV,VE,VP
  DCM : Outport  VectorParamsAs1DForOutWhenUnconnected=off
  Euler : Outport  Port=2  VectorParamsAs1DForOutWhenUnconnected=off
  wires:
  Rotation Angles to Direction Cosine Matrix/1 -> DCM/1
  "p q r "/1 -> phidot thetadot psidot/1
  Discrete-Time Integrator3/1 -> Euler/1, Selector/1, phidot thetadot psidot/2
  Selector/1 -> Rotation Angles to Direction Cosine Matrix/1
  phidot thetadot psidot/1 -> Discrete-Time Integrator3/1

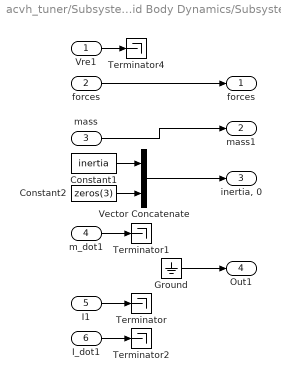
== system acvh_tuner/Subsystem/6DOF Rigid Body Dynamics/Subsystem1 ==
  Vre1 : Inport
  forces : Inport  Port=2
  "mass " : Inport  Port=3
  m_dot1 : Inport  Port=4  OutDataTypeStr=double
  I1 : Inport  Port=5  OutDataTypeStr=double
  I_dot1 : Inport  Port=6  OutDataTypeStr=double
  Constant1 : Constant  Value=inertia  OutDataTypeStr=Inherit: Inherit via back propagation
  Constant2 : Constant  Value=zeros(3)
  Ground : Ground
  Terminator{,1..2,4} (4 alike) : Terminator
  Vector Concatenate : Concatenate  Mode=Multidimensional array
  "forces " : Outport  VectorParamsAs1DForOutWhenUnconnected=off
  mass1 : Outport  Port=2  VectorParamsAs1DForOutWhenUnconnected=off
  "inertia, 0" : Outport  Port=3  VectorParamsAs1DForOutWhenUnconnected=off
  Out1 : Outport  Port=4  VectorParamsAs1DForOutWhenUnconnected=off
  wires:
  Constant2/1 -> Vector Concatenate/2
  Constant1/1 -> Vector Concatenate/1
  I1/1 -> Terminator/1
  I_dot1/1 -> Terminator2/1
  forces/1 -> "forces "/1
  Vector Concatenate/1 -> "inertia, 0"/1
  Ground/1 -> Out1/1
  m_dot1/1 -> Terminator1/1
  Vre1/1 -> Terminator4/1
  "mass "/1 -> mass1/1

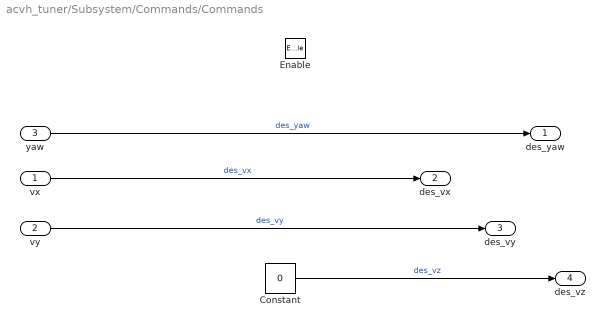
== system acvh_tuner/Subsystem/Commands/Commands  ==
  vx : Inport
  vy : Inport  Port=2
  yaw : Inport  Port=3
  Enable : EnablePort
  Constant : Constant  Value=0
  des_yaw : Outport
  des_vx : Outport  Port=2
  des_vy : Outport  Port=3
  des_vz : Outport  Port=4
  wires:
  vy/1 -> des_vy/1  "des_vy"
  vx/1 -> des_vx/1  "des_vx"
  Constant/1 -> des_vz/1  "des_vz"
  yaw/1 -> des_yaw/1  "des_yaw"

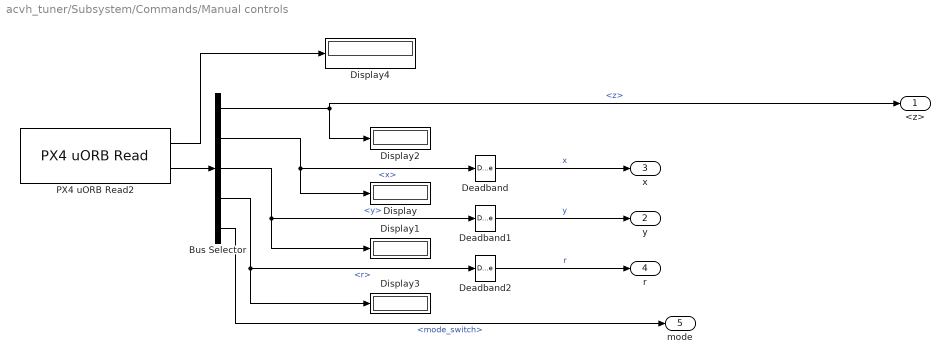
== system acvh_tuner/Subsystem/Commands/Manual controls ==
  Bus Selector : BusSelector  OutputSignals=z,x,y,r,mode_switch
  Deadband : DeadZone  LowerValue=-0.05  UpperValue=0.05  SaturateOnIntegerOverflow=on
  Deadband1 : DeadZone  LowerValue=-0.05  UpperValue=0.05  SaturateOnIntegerOverflow=on
  Deadband2 : DeadZone  LowerValue=-0.05  UpperValue=0.05  SaturateOnIntegerOverflow=on
  Display{,1..4} (5 alike) : Display
  PX4 uORB Read2 : px4uORBlib/PX4 uORB Read  uORBTopic=manual_control_setpoint  selectInstance=manual_control_setpoint  SampleTime=SampleTime  BlockingMode=off  BlockTimeout=1e-3
      settings: SourceProductBaseCode=PX4AUTOPILOTS
  <z> : Outport
  y : Outport  Port=2
  x : Outport  Port=3
  r : Outport  Port=4
  mode : Outport  Port=5
  wires:
  Deadband1/1 -> y/1  "y"
  PX4 uORB Read2/2 -> Bus Selector/1
  Bus Selector/1 -> Display2/1, <z>/1  "<z>"
  Bus Selector/2 -> Display/1, Deadband/1  "<x>"
  PX4 uORB Read2/1 -> Display4/1
  Deadband2/1 -> r/1  "r"
  Deadband/1 -> x/1  "x"
  Bus Selector/3 -> Display1/1, Deadband1/1  "<y>"
  Bus Selector/4 -> Display3/1, Deadband2/1  "<r>"
  Bus Selector/5 -> mode/1  "<mode_switch>"

== matlab function acvh_tuner/MATLAB Function ==
  data: tuned input; y output; z input
function y = fcn(tuned, z)
    temp = 0;
    if(z<-6)
       temp = -.08;
    end
    if(z>-4)
        temp = .08;
    end 
y = temp;

== matlab function acvh_tuner/Force and Moment Calculation/Aerodynamic drag/calcDragVector ==
  data: airVel input; dragVec output; dragCoeff input
function dragVec = fcn(airVel, dragCoeff)

dragVec = dragCoeff * norm(airVel) * airVel;

end

== matlab function acvh_tuner/Altitude > 0 Constraint ==
  data: Ve input; Xe input; Xe output; Vb output; DCM_be input; omega_b input; omega_b_nav output
function [Xe, Vb, omega_b_nav] = fcn(Ve, Xe, DCM_be, omega_b)
z = Xe(3);
Vz = Ve(3);

if z>=0 && Vz >= 0 %drone on or below gnd and still trying to do down
    Ve = Ve*0; %reset velocity
    omega_b = omega_b*0; %reset omega
    z = 0; % reset height
    Xe(3) = z;
end
Ve(3) = 0;

Vb = Ve;
omega_b_nav = DCM_be'*omega_b;
end

== matlab function acvh_tuner/Force and Moment Calculation/Rotor Model/MATLAB Function ==
  data: thrustEachRotor input; tauEachRotor input; rotorPositions input; netF output; netM output; rotorDir input
function [netF, netM] = getForceMoment(thrustEachRotor, tauEachRotor, rotorPositions, rotorDir)
%#codegen
Fx = 0;
Fy = 0;
Fz = -sum(thrustEachRotor);

netF = [Fx; Fy; Fz];

netM = [0; 0; 0]; %initialize
    for i = 1:4
        rotPos = rotorPositions(:, i);
        Fi = [0, 0, -thrustEachRotor(i)]';
        netM = netM +  cross(rotPos, Fi);%contribution from thrusts of each propeller
        netM(3) = netM(3) - rotorDir(i)*tauEachRotor(i); %contribution from counter torque acting on propeller
    end

end
